simulink model "yaw"  (R2020b)
settings: Solver=VariableStepAuto  StartTime=0.0  StopTime=10.0  RelTol=1e-3
values from neighbouring files (symbols this model uses):
  Cwy1 = 1144.7    [Calculations.m]
  Cwy2 = 22.52    [Calculations.m]
  Jyy = 366    [Calculations.m]
  k1_yaw = (M^2 + M* sqrt(M^2 - 1)) / ( 4 * T_omega * K_omega * kc)    [Calculations.m]
  k2_yaw = ( T_propulsion_x*(Jyy+lambda55) - (2*Cwy1 * w_linearization + Cwy2)* T_omega^2) /     ( T_omega^2 * kc * K_propulsion_w )    (= 0.636961631851)    [Calculations.m]
  K_thruster = P1 / U1    (= 24.525)    [Calculations.m]
  kc = 57.2958    [Calculations.m]    (also in Parameters_2.m)
  l = 0.225    [Calculations.m]
  lambda55 = 117.08    [Calculations.m]
  T_thruster = 0.3    [Calculations.m]
libraries: slctrlblks x1
settings Model: Creator=corsair  LastModifiedBy=corsair

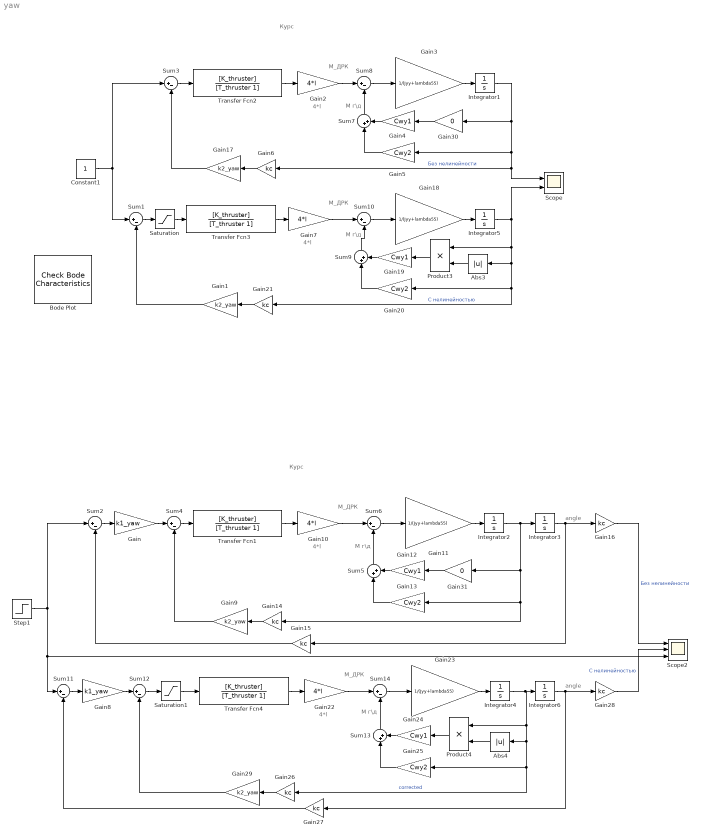
== system yaw ==
  note: M_ДРК
  note: 4*l
  note: angle
  note: Курс
  note: M г\д
  note: M_ДРК
  note: 4*l
  note: Курс
  note: M г\д
  note: M_ДРК
  note: 4*l
  note: M г\д
  note: M_ДРК
  note: 4*l
  note: angle
  note: M г\д
  Abs3 : Abs
  Abs4 : Abs
  Bode Plot : slctrlblks/Model Verification/Check Bode  Characteristics  InstantiateOnLoad=on  SaveOperatingPoints=off  LinearizationIOs={'/Constant1', 1, 'in', 'on', '';'/Integrator1', 1, 'out', 'on', ''}  LinearizeAt=SnapshotTimes  SnapshotTimes=[0]  TriggerType=rising  SampleTime=auto  RateConversionMethod=zoh  PreWarpFreq=10  UseExactDelayModel=off  UseFullBlockNameLabels=off  UseBusSignalLabels=off  enabled=on  stopWhenAssertionFail=off  export=off  ViewDlgPos=[1 1 1117 626]  OpenViewOnLoad=off  LaunchViewOnOpen=on  FrequencyUnits=rad/s  MagnitudeUnits=dB  PhaseUnits=deg  TimeUnits=seconds  EnableUpperBound=off  UpperBoundFrequencies=[]  UpperBoundMagnitudes=[]  EnableLowerBound=off  LowerBoundFrequencies=[]  LowerBoundMagnitudes=[]
  Constant1 : Constant
  Gain : Gain  Gain=k1_yaw
  Gain{1,9,17,29} (4 alike) : Gain  Gain=k2_yaw
  Gain{2,7,10,22} (4 alike) : Gain  Gain=4*l
  Gain{3,11,18,23} (4 alike) : Gain  Gain=1/(Jyy+lambda55)
  Gain{4,12,19,24} (4 alike) : Gain  Gain=Cwy1
  Gain{5,13,20,25} (4 alike) : Gain  Gain=Cwy2
  Gain{6,14..16,21,26..28} (8 alike) : Gain  Gain=kc
  Gain30 : Gain  Gain=0
  Gain31 : Gain  Gain=0
  Gain8 : Gain  Gain=k1_yaw
  Integrator{1..6} (6 alike) : Integrator
  Product3 : Product
  Product4 : Product
  Saturation : Saturate  UpperLimit=24  LowerLimit=-24
  Saturation1 : Saturate  UpperLimit=24  LowerLimit=-24
  Scope : Scope  NumInputPorts=2
  Scope2 : Scope  NumInputPorts=3
  Step1 : Step  SampleTime=0
  Sum{1..4,6,8,10..12,14} (10 alike) : Sum  Inputs=|+-
  Sum{5,7,9,13} (4 alike) : Sum  Inputs=|++
  Transfer Fcn{1..4} (4 alike) : TransferFcn  Numerator=[K_thruster]  Denominator=[T_thruster 1]
  wires:
  Sum6/1 -> Gain11/1
  Transfer Fcn1/1 -> Gain10/1
  Gain11/1 -> Integrator2/1
  Sum5/1 -> Sum6/2
  Sum4/1 -> Transfer Fcn1/1
  Gain16/1 -> Scope2/1  "Без нелинейности"
  Gain14/1 -> Gain9/1
  Integrator3/1 -> Gain16/1, Gain15/1
  Sum2/1 -> Gain/1
  Integrator2/1 -> Integrator3/1, Gain31/1, Gain14/1, Gain13/1
  Gain9/1 -> Sum4/2
  Gain31/1 -> Gain12/1
  Gain15/1 -> Sum2/2
  Gain13/1 -> Sum5/1
  Gain/1 -> Sum4/1
  Gain10/1 -> Sum6/1
  Gain12/1 -> Sum5/2
  Gain4/1 -> Sum7/2
  Gain2/1 -> Sum8/1
  Constant1/1 -> Sum3/1, Sum1/1
  Gain5/1 -> Sum7/1
  Gain30/1 -> Gain4/1
  Gain17/1 -> Sum3/2
  Integrator1/1 -> Scope/1, Gain6/1, Gain5/1, Gain30/1  "Без нелинейности"
  Gain6/1 -> Gain17/1
  Sum3/1 -> Transfer Fcn2/1
  Sum7/1 -> Sum8/2
  Gain3/1 -> Integrator1/1
  Transfer Fcn2/1 -> Gain2/1
  Sum8/1 -> Gain3/1
  Sum10/1 -> Gain18/1
  Transfer Fcn3/1 -> Gain7/1
  Gain18/1 -> Integrator5/1
  Sum9/1 -> Sum10/2
  Abs3/1 -> Product3/2
  Gain21/1 -> Gain1/1
  Integrator5/1 -> Scope/2, Gain21/1, Gain20/1, Abs3/1, Product3/1  "С нелинейностью"
  Gain1/1 -> Sum1/2
  Product3/1 -> Gain19/1
  Gain20/1 -> Sum9/1
  Gain7/1 -> Sum10/1
  Gain19/1 -> Sum9/2
  Saturation/1 -> Transfer Fcn3/1
  Sum1/1 -> Saturation/1
  Gain24/1 -> Sum13/2
  Gain22/1 -> Sum14/1
  Gain8/1 -> Sum12/1
  Gain25/1 -> Sum13/1
  Gain27/1 -> Sum11/2
  Product4/1 -> Gain24/1
  Gain29/1 -> Sum12/2
  Integrator4/1 -> Gain26/1, Gain25/1, Abs4/1, Product4/1, Integrator6/1  "corrected"
  Sum11/1 -> Gain8/1
  Integrator6/1 -> Gain27/1, Gain28/1
  Gain26/1 -> Gain29/1
  Abs4/1 -> Product4/2
  Step1/1 -> Sum11/1, Scope2/3, Sum2/1
  Gain28/1 -> Scope2/2  "С нелинейностью"
  Sum13/1 -> Sum14/2
  Gain23/1 -> Integrator4/1
  Transfer Fcn4/1 -> Gain22/1
  Sum14/1 -> Gain23/1
  Sum12/1 -> Saturation1/1
  Saturation1/1 -> Transfer Fcn4/1
